simulink model "Ready_to_deploy"  (R2020a)
settings: Solver=FixedStepDiscrete  StartTime=0.0  StopTime=Inf  FixedStep=1e-4  MaxStep=1e-4  RelTol=1e-3  EnableMultiTasking=on
values from neighbouring files (symbols this model uses):
  parameter =     [parameter.mat]
libraries: c2802xlib x2, idelinklib_common x2, dspsigops x2, powerlib_meascontrol x1
settings Model: ExtModeTrigDuration=8  Creator=ibrahim yosry  LastModifiedBy=ibrahim yosry
settings SolverCC: InitialStep=1e-4  AutoInsertRateTranBlk=on
settings OptimizationCC: DefaultUnderspecifiedDataType=single  EnhancedBackFolding=on  PassReuseOutputArgsAs=Individual arguments  MaxStackSize=1024  OptimizeBlockOrder=speed  DifferentSizesBufferReuse=on  OptimizationCustomize=off  DenormalBehavior=FlushToZero  EfficientTunableParamExpr=on
settings DebuggingCC: ParameterTunabilityLossMsg=error
settings HardwareCC: ProdBitPerChar=16  ProdBitPerInt=16  ProdBitPerPointer=32  ProdBitPerSizeT=32  ProdBitPerPtrDiffT=32  ProdLargestAtomicInteger=Integer  ProdLargestAtomicFloat=None  ProdWordSize=16  ProdLongLongMode=on  ProdHWDeviceType=Texas Instruments->C2000
settings SFSimCC: MATLABDynamicMemAlloc=off
settings RTWCC: SystemTargetFile=ert.tlc  HardwareBoard=TI Delfino F28379D LaunchPad  TLCOptions=-aInlineSetEventsForThisBaseRateFcn=TLC_FALSE -aSuppressMultiTaskScheduler=TLC_FALSE -aRateBasedStepFcn=1  TemplateMakefile=ert_default_tmf  Toolchain=Texas Instruments Code Composer Studio (C2000)
settings CodeAppCC: ForceParamTrailComments=on  IgnoreCustomStorageClasses=off  OperatorAnnotations=on  SimulinkDataObjDesc=on  SFDataObjDesc=on  InsertBlockDesc=on
settings ERTTargetCC: CodeReplacementLibrary=TI C28x  SupportVariableSizeSignals=on  ExtModeStaticAllocSize=10000

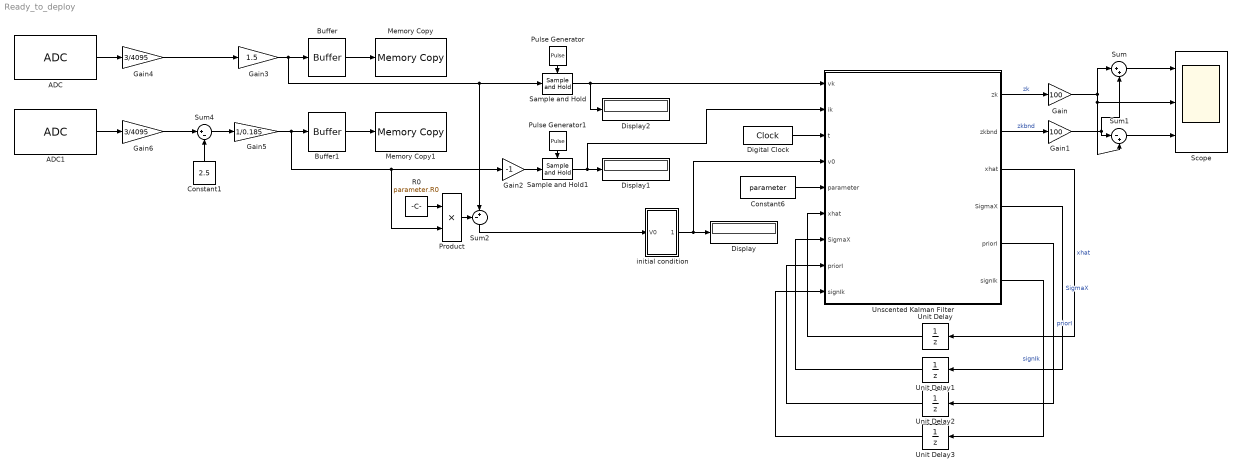
== system Ready_to_deploy ==
  ADC : c2802xlib/ADC  blkParamProc=C2000_Type4  ADCModule=A  samplingMode=Single sample mode  ADCResolution=12-bit (Single-ended input)  useSOC1=SOC0  useSOC2=SOC0_SOC1  SOCAcquisitionWindow=15  SOCTriggerSource=Software  SOCInterruptTrigger=No ADCINT  Ts=0.001  dType=double  postInterrupt=off  interruptSel=ADCINT1  ADCINTContinuous=on  endma=off  chdma=1  conv1=ADCINA0  conv2=ADCINA0 and ADCINB0  conv1_Type4=ADCIN3  conv2_Type4=ADCIN0 and ADCIN1
  ADC1 : c2802xlib/ADC  blkParamProc=C2000_Type4  ADCModule=C  samplingMode=Single sample mode  ADCResolution=12-bit (Single-ended input)  useSOC1=SOC0  useSOC2=SOC0_SOC1  SOCAcquisitionWindow=15  SOCTriggerSource=Software  SOCInterruptTrigger=No ADCINT  Ts=0.001  dType=double  postInterrupt=off  interruptSel=ADCINT1  ADCINTContinuous=on  endma=off  chdma=1  conv1=ADCINA0  conv2=ADCINA0 and ADCINB0  conv1_Type4=ADCIN2  conv2_Type4=ADCIN0 and ADCIN1
  Buffer : Buffer  N=500  OutputFrames=off
  Buffer1 : Buffer  N=500  OutputFrames=off
  Constant1 : Constant  Value=2.5  SampleTime=1e-1
  Constant6 : Constant  Value=parameter  VectorParams1D=off  OutDataTypeStr=Bus: parameter_bus  SampleTime=1e-1
  Digital Clock : DigitalClock  SampleTime=1e-1
  Display : Display
  Display1 : Display
  Display2 : Display
  Gain : Gain  Gain=100
  Gain1 : Gain  Gain=100
  Gain2 : Gain  Gain=-1
  Gain3 : Gain  Gain=1.5
  Gain4 : Gain  Gain=3/4095
  Gain5 : Gain  Gain=1/0.185
  Gain6 : Gain  Gain=3/4095
  Memory Copy : idelinklib_common/Memory Copy  copyFrom=Input port  copyFromAddressSource=Specify via dialog  copyFromAddress=hex2dec('00001000')  copyFromSrcCode=myVariableSrc  dataTypeFrom=Inherit from input port  dataDimensionFrom=500  useOffsetFrom=off  offsetFromSrc=Specify via dialog  offsetFrom=0  strideFrom=1  copyTo=Specified address  copyToAddressSource=Specify via dialog  copyToAddress=hex2dec('00002000')  copyToSrcCode=myVariableDst  dataTypeTo=double  useOffsetTo=off  offsetToSrc=Specify via dialog  offsetTo=0  strideTo=1  sampleTime=inf  useInitValue=off  initValueSrc=Specify constant value  initValue=1  initValueSrcCode=myInitValueVariable  useAsMask=off  maskOperator=bitwise AND  useTermValue=off  termValue=1  isRealtimeEnabled=off  emitCCBeforeWrite=off  CCBeforeWrite=/* Custom Code Before Write*/  emitCCAfterWrite=off  CCAfterWrite=/* Custom Code After Write*/  useDMACopy=off  enableBlockingMode=off
      settings: SourceProductBaseCode=ME
  Memory Copy1 : idelinklib_common/Memory Copy  copyFrom=Input port  copyFromAddressSource=Specify via dialog  copyFromAddress=hex2dec('00001000')  copyFromSrcCode=myVariableSrc  dataTypeFrom=Inherit from input port  dataDimensionFrom=500  useOffsetFrom=off  offsetFromSrc=Specify via dialog  offsetFrom=0  strideFrom=1  copyTo=Specified address  copyToAddressSource=Specify via dialog  copyToAddress=hex2dec('00002000')  copyToSrcCode=myVariableDst  dataTypeTo=double  useOffsetTo=off  offsetToSrc=Specify via dialog  offsetTo=0  strideTo=1  sampleTime=inf  useInitValue=off  initValueSrc=Specify constant value  initValue=1  initValueSrcCode=myInitValueVariable  useAsMask=off  maskOperator=bitwise AND  useTermValue=off  termValue=1  isRealtimeEnabled=off  emitCCBeforeWrite=off  CCBeforeWrite=/* Custom Code Before Write*/  emitCCAfterWrite=off  CCAfterWrite=/* Custom Code After Write*/  useDMACopy=off  enableBlockingMode=off
      settings: SourceProductBaseCode=ME
  Product : Product
  Pulse Generator : DiscretePulseGenerator  PulseType=Time based  Period=1e-1  PulseWidth=5
  Pulse Generator1 : DiscretePulseGenerator  PulseType=Time based  Period=1e-1  PulseWidth=5
  R0 : Constant  Value=parameter.R0  SampleTime=1e-1
  Sample and Hold : dspsigops/Sample and Hold  trig=Rising edge  initCond=0  latchinput=off
  Sample and Hold1 : dspsigops/Sample and Hold  trig=Rising edge  initCond=0  latchinput=off
  Scope : Scope  NumInputPorts=3
  Sum : Sum  Inputs=|++
  Sum1 : Sum  Inputs=|-+
  Sum2 : Sum  Inputs=-+|
  Sum4 : Sum  Inputs=|+-
  Unit Delay : UnitDelay  InitialCondition=[1;0;0]  SampleTime=1e-1  StateName=xhat  HasFrameUpgradeWarning=on
  Unit Delay1 : UnitDelay  InitialCondition=diag([1e-6 1e-8 2e-4])  SampleTime=1e-1  StateName=SigmaX  HasFrameUpgradeWarning=on
  Unit Delay2 : UnitDelay  SampleTime=1e-1  StateName=priorI  HasFrameUpgradeWarning=on
  Unit Delay3 : UnitDelay  SampleTime=1e-1  StateName=signIk  HasFrameUpgradeWarning=on
  Unscented Kalman Filter : MATLAB Function  TreatAsAtomicUnit=on
  initial condition : Subsystem
      mask Display: image('F:\hima\zpEWIvRg.jpg'); % Use "Edit Image" on toolstrip to change.
  wires:
  Unscented Kalman Filter/3(xhat) -> Unit Delay/1  "xhat"
  Unscented Kalman Filter/1(zk) -> Gain/1  "zk"
  Unscented Kalman Filter/2(zkbnd) -> Gain1/1  "zkbnd"
  Gain1/1 -> Sum/2, Sum1/1
  Gain/1 -> Sum/1, Sum1/2, Scope/2
  Sum/1 -> Scope/1
  Sum1/1 -> Scope/3
  initial condition/1(Out1) -> Display/1, Unscented Kalman Filter/4(v0)
  Unit Delay/1 -> Unscented Kalman Filter/6("xhat ")
  Pulse Generator/1 -> Sample and Hold/Trigger
  Pulse Generator1/1 -> Sample and Hold1/Trigger
  Sample and Hold1/1 -> Unscented Kalman Filter/2(ik), Display1/1
  Constant6/1 -> Unscented Kalman Filter/5(parameter)
  Digital Clock/1 -> Unscented Kalman Filter/3(t)
  Unscented Kalman Filter/4(SigmaX) -> Unit Delay1/1  "SigmaX"
  Unscented Kalman Filter/5(priorI) -> Unit Delay2/1  "priorI"
  Unscented Kalman Filter/6(signIk) -> Unit Delay3/1  "signIk"
  Unit Delay3/1 -> Unscented Kalman Filter/9("signIk ")
  Unit Delay2/1 -> Unscented Kalman Filter/8("priorI ")
  Unit Delay1/1 -> Unscented Kalman Filter/7("SigmaX ")
  Gain5/1 -> Product/2, Gain2/1, Buffer1/1
  Gain2/1 -> Sample and Hold1/1
  R0/1 -> Product/1
  Product/1 -> Sum2/1
  Gain3/1 -> Sum2/2, Sample and Hold/1, Buffer/1
  Sum2/1 -> initial condition/1(V0)
  Sample and Hold/1 -> Unscented Kalman Filter/1(vk), Display2/1
  Gain4/1 -> Gain3/1
  ADC/1 -> Gain4/1
  Buffer/1 -> Memory Copy/1
  Buffer1/1 -> Memory Copy1/1
  ADC1/1 -> Gain6/1
  Constant1/1 -> Sum4/2
  Sum4/1 -> Gain5/1
  Gain6/1 -> Sum4/1

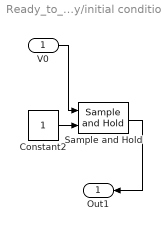
== system Ready_to_deploy/initial condition ==
  V0 : Inport
  Constant2 : Constant  SampleTime=1e-1
  Sample and Hold : powerlib_meascontrol/Additional Components/Sample and Hold  ic=0  Ts=3600
      settings: SourceProductBaseCode=PS
  Out1 : Outport  VectorParamsAs1DForOutWhenUnconnected=off
  wires:
  Constant2/1 -> Sample and Hold/2
  V0/1 -> Sample and Hold/1
  Sample and Hold/1 -> Out1/1

== matlab function Ready_to_deploy/Unscented Kalman Filter ==
  settings: updateMethod=DISCRETE  sampleTime=1e-1
  data: vk input; zk output; ik input; t input; v0 input; parameter input; xhat input double; zkbnd output; xhat output; SigmaX input double; priorI input double; signIk input double; SigmaX output; priorI output; signIk output
function [zk,zkbnd,xhat,SigmaX,priorI,signIk] = iterSPKF(vk,ik,t,v0,parameter,xhat,SigmaX,priorI,signIk)
parameter.deltat=1e-1;
SigmaX0 = diag([1e-6 1e-8 2e-4]);
SigmaV = 2e-1;
SigmaW = 2e-1;
Snoise = chol(blkdiag(SigmaW,SigmaV),'lower');
irk0 = 0;
hk0 = 0;
zkInd = 1;
irkInd = 2;
hkInd = 3;
ocv=parameter.ocv;
soc=parameter.soc;
Nx = 3;
Nw = 1;
Nv = 1;
Na = Nx+Nw+Nv;
h = sqrt(3);
alpha1 = (h*h-Na)/(h*h);
alpha2 = 1/(2*h*h);
alpham = [alpha1; alpha2*ones(2*Na,1)];
alphac = alpham;
RC      = parameter.RC;
G       = parameter.G;
Q       = parameter.Q;
deltat  = parameter.deltat;
R0      = parameter.R0;
R       = parameter.R;
M0      = parameter.M0;
M       = parameter.M;
zkInd   = parameter.zkInd;
irkInd  = parameter.irkInd;
hkInd   = parameter.hkInd;

eta     = 1;
if ik<0 
ik=ik*eta;
end

if t<1e-4
j1=find(min(abs(ocv-v0))==abs(ocv-v0));
j=j1(1,:);
SOC0 = soc(j);
xhat = [SOC0;irk0;hk0];
SigmaX = SigmaX0;
priorI = 0;
signIk = 0;
end

I       =  priorI;
if abs(ik)>Q/100
signIk = sign(ik);
end
xhata = [xhat; zeros([Nw+Nv 1])];
sigmaXa = chol(SigmaX,'lower');
sigmaXa= blkdiag(sigmaXa,Snoise);
Xa = xhata(:,ones([1 2*Na+1])) + h*[zeros([Na 1]),sigmaXa,-sigmaXa];
Xx = stateEqn(Xa(1:Nx,:),I,Xa(Nx+1:Nx+Nw,:),parameter);
xhat = Xx*alpham;
Xs = Xx - xhat(:,ones([1 2*Na+1]));
SigmaX = Xs*diag(alphac)*Xs';
I = ik;
yk = vk;
Y = outputEqn(Xx,I,Xa(5,:),signIk,parameter);
yhat = Y*alpham;
Ys = Y - yhat(:,ones([1 2*Na+1]));
SigmaXY = Xs*diag(alphac)*Ys';
SigmaY = Ys*diag(alphac)*Ys';
L = SigmaXY/SigmaY;
ytelda = yk - yhat;
xhat = xhat + L*ytelda;
xhat(hkInd) = min(0.99,max(-0.99,xhat(hkInd)));
SigmaX = SigmaX - L*SigmaY*L';
priorI = ik;
zk = xhat(zkInd);
zkbnd = 3*sqrt(SigmaX(zkInd,zkInd));
function xnew = stateEqn(xold,current,xnoise,parameter)
current = current + xnoise;
RC      = parameter.RC;
G       = parameter.G;
Q       = parameter.Q;
deltat  = parameter.deltat;
zkInd   = parameter.zkInd;
irkInd  = parameter.irkInd;
hkInd   = parameter.hkInd;
Ah = exp(-abs(current*G*deltat/(3600*Q)));
xnew = 0*xold;
xnew(irkInd,:) = RC*xold(irkInd,:) + (1-RC)*current;
xnew(hkInd,:) = Ah.*xold(hkInd,:) + (Ah-1).*sign(current);
xnew(zkInd,:) = xold(zkInd,:) - current*deltat/(3600*Q);
end
function y = outputEqn(x,current,ynoise,signIk,parameter)
soc     = parameter.soc;
ocv     = parameter.ocv;
R0      = parameter.R0;
R       = parameter.R;
M0      = parameter.M0;
M       = parameter.M;
zkInd   = parameter.zkInd;
irkInd  = parameter.irkInd;
hkInd   = parameter.hkInd;
i = zeros(11,1);
for k=1:11
i2=find(min(abs(soc-x(zkInd,k)*ones(length(soc),1)))==abs(soc-x(zkInd,k)*ones(length(soc),1)));
i2(1)=min(1,max(length(soc),i2(1)));
i(k,1)=i2(1,1);
end
y = ocv(i)' - R * x(irkInd,:) - R0 * current + M * x(hkInd,:) + M0 * signIk + ynoise;
end
end
